simulink model "Task29"  (R2022b)
settings: Solver=VariableStepAuto  StartTime=0.0  StopTime=10.0  RelTol=1e-3
settings Model: Creator=LOQ  LastModifiedBy=LOQ
settings OptimizationCC: ReuseModelBlockBuffer=on
settings RTWCC: GPUComputeCapability=5.0
settings ConfigComp: CovBoundaryAbsTol=1.0e-5

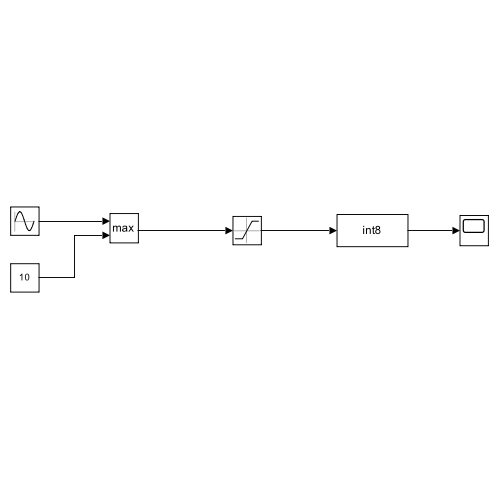
[thumbnail: Simulink's stored preview of the top-level diagram]
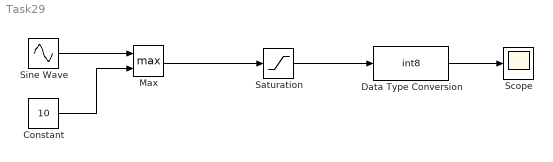
== system Task29 ==
  Constant : Constant  Value=10
  Data Type Conversion : DataTypeConversion  OutDataTypeStr=int8  SaturateOnIntegerOverflow=off  RndMeth=Floor
  Max : MinMax  Function=max  Inputs=2
  Saturation : Saturate  UpperLimit=90  LowerLimit=0
  Scope : Scope
  Sine Wave : Sin  Amplitude=100  SampleTime=0
  wires:
  Constant/1 -> Max/2
  Sine Wave/1 -> Max/1
  Max/1 -> Saturation/1
  Saturation/1 -> Data Type Conversion/1
  Data Type Conversion/1 -> Scope/1
